simulink model "lab_5"  (R2021a)
settings: Solver=FixedStepAuto  StartTime=0.0  StopTime=10  FixedStep=0.01  RelTol=1e-3
settings Model: Creator=fantavit  LastModifiedBy=fantavit

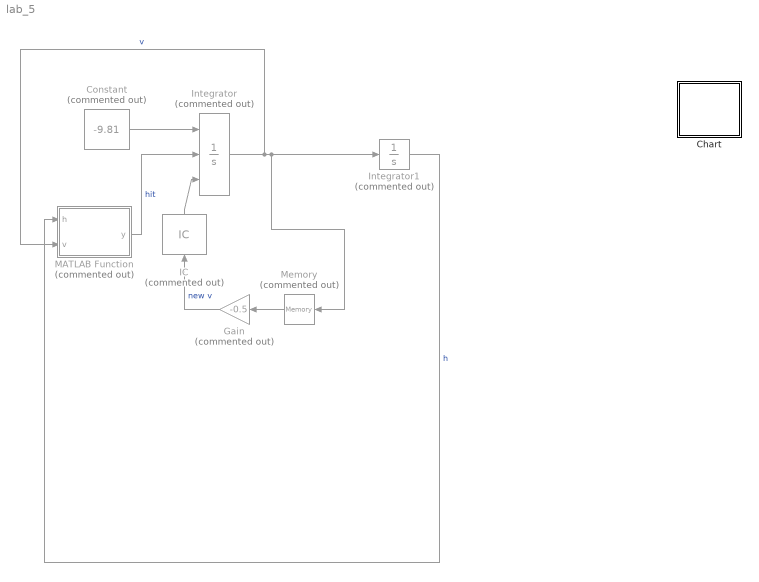
== system lab_5 ==
  Chart : Stateflow chart  TreatAsAtomicUnit=on
  Constant : Constant  Commented=on  Value=-9.81
  Gain : Gain  Commented=on  Gain=-0.5
  IC : InitialCondition  Commented=on  Value=0
  Integrator : Integrator  Commented=on  ExternalReset=falling  InitialConditionSource=external
  Integrator1 : Integrator  Commented=on  InitialCondition=10
  MATLAB Function : MATLAB Function  Commented=on  TreatAsAtomicUnit=on
  Memory : Memory  Commented=on
  wires:
  Integrator/1 -> MATLAB Function/2(v), Memory/1, Integrator1/1  "v"
  Integrator1/1 -> MATLAB Function/1(h)  "h"
  Constant/1 -> Integrator/1
  MATLAB Function/1(y) -> Integrator/2  "hit"
  Gain/1 -> IC/1  "new v"
  IC/1 -> Integrator/3
  Memory/1 -> Gain/1

== stateflow chart lab_5/Chart ==
  state Ball
  (default) -> Ball
  Ball -> Ball : [h <= 0, v < 0
      | ]{v = -0.5*v}
  data: h local; v local

== matlab function lab_5/MATLAB Function ==
  data: h input; y output; v input
function y = fcn(h, v)
y = (h > 0) || ((abs(h) < eps) && (v >= 0));
% y = (h <= 0) && (v < 0);
